simulink model "generic_truck"  (R2025a)
settings: Solver=VariableStepAuto  StartTime=0.0  StopTime=600  FixedStep=0.01  MaxStep=0.001  RelTol=1e-3  EnableMultiTasking=on
libraries: TruckMaker4SL x205, simulink x1
(part 1 of 9)
settings Model: ModifiedByFormat=IPG  SimulationMode=accelerator  NumberOfSteps=10  ExtModeAutoUpdateStatusClock=off  Creator=IPG  LastModifiedBy=IPG
settings SolverCC: AlgebraicLoopSolver=TrustRegion
settings DataIOCC: LimitDataPoints=on  SaveFormat=Array  SignalLoggingSaveFormat=ModelDataLogs  ReturnWorkspaceOutputs=off  SignalLoggingName=sigsOut
settings OptimizationCC: BooleanDataType=off  ReuseModelBlockBuffer=off  ExpressionDepthLimit=2147483647.0  InitFltsAndDblsToZero=on  LifeSpan=inf
settings DebuggingCC: SaveWithParameterizedLinksMsg=none  UnderspecifiedInitializationDetection=Classic  MergeDetectMultiDrivingBlocksExec=none  SignalResolutionControl=TryResolveAllWithWarning  MultiTaskDSMMsg=warning  MultiTaskCondExecSysMsg=none  FcnCallInpInsideContextMsg=warning  UnconnectedInputMsg=warning  UnconnectedOutputMsg=warning  UnconnectedLineMsg=warning  StateNameClashWarn=warning  SFUnexpectedBacktrackingDiag=warning  SFNoUnconditionalDefaultTransitionDiag=warning  ArithmeticOperatorsInVariantConditions=warning
settings HardwareCC: ProdBitPerPointer=32.0  ProdBitPerSizeT=32.0  ProdBitPerPtrDiffT=32.0  ProdLargestAtomicFloat=None  ProdIntDivRoundTo=Undefined  ProdEndianess=Unspecified  ProdWordSize=32.0  ProdHWDeviceType=32-bit Generic  TargetUnknown=on
settings ModelReferenceCC: EnableRefExpFcnMdlSchedulingChecks=on  PropagateSignalLabelsOutOfModel=off
settings SFSimCC: SimUseLocalCustomCode=off  CustomCodeUndefinedFunction=UseInterfaceOnly
settings RTWCC: RTWUseLocalCustomCode=off  GPUComputeCapability=3.5  DLArmComputeVersion=19.05
settings CodeAppCC: MaxIdLength=63.0  StateflowObjectComments=on
settings GRTTargetCC: TargetFcnLib=ansi_tfl_tmw.mat  TargetLangStandard=C89/C90 (ANSI)  CombineOutputUpdateFcns=off  GRTInterface=on
settings ConfigComp: CovMetricSettings=dw  CovSaveCumulativeToWorkspaceVar=on  CovSaveSingleToWorkspaceVar=on  CovExternalEMLEnable=off

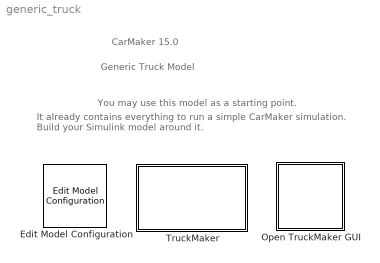
== system generic_truck ==
  note: Generic Truck Model
  note: CarMaker 15.0
  note: You may use this model as a starting point.
  note: It already contains everything to run a simple CarMaker simulation.
      | Build your Simulink model around it.
  Edit Model Configuration : TruckMaker4SL/Edit Model Configuration  SFunctionModules=''
      settings: SourceProductName=TruckMaker4SL
  Open TruckMaker GUI : Subsystem  LoadFcn=if ~length(which('cmself')), cmenv; end
      settings: OpenFcn=cmblockmagic('gui_fix_display'); TM_Simulink
      mask Display: image(imread('TruckMakerGUI.png'));
  TruckMaker : Subsystem  TreatAsAtomicUnit=on
      mask Display: image(imread('TruckMakerSys.png'));

== system generic_truck/Open TruckMaker GUI ==
  S-Function : S-Function  FunctionName=cm_gui  SFunctionDeploymentMode=off  EnableBusSupport=off

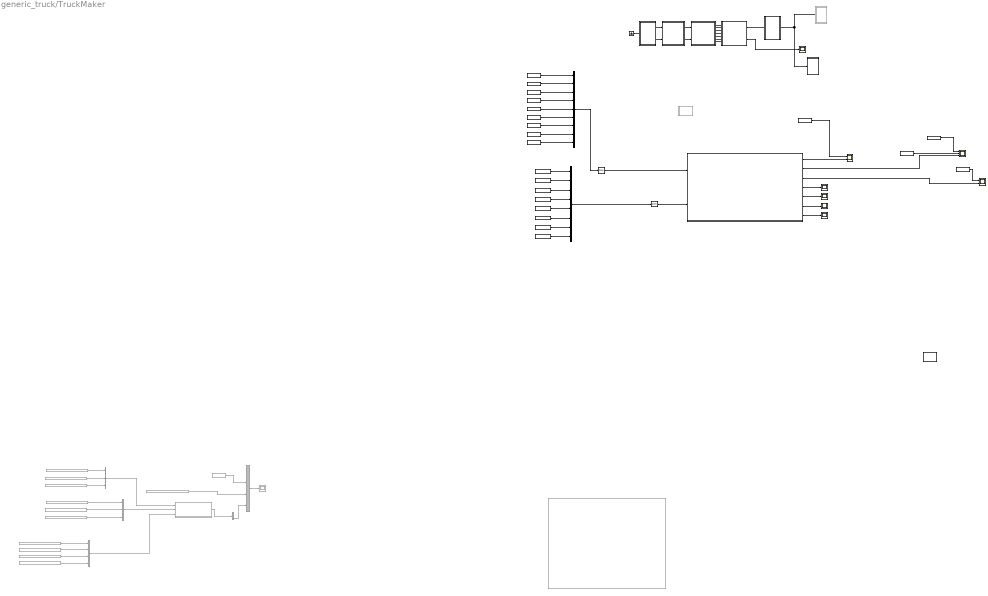
== system generic_truck/TruckMaker ==
  ACC_X : TruckMaker4SL/Read CM Dict  xname=Sensor.Inertial.Vhcl.VchBdy.Acc_B.x  xsync=off  xstime=Continuous
      settings: SourceProductName=TruckMaker4SL
  ACC_Y : TruckMaker4SL/Read CM Dict  xname=Sensor.Inertial.Vhcl.VchBdy.Acc_B.y  xsync=off  xstime=Continuous
      settings: SourceProductName=TruckMaker4SL
  CM_FIRST : Subsystem
  CM_LAST : Subsystem
  "Comparison Block Forces " : Subsystem  Commented=on
  CyFL : Scope
      settings: ActiveDisplayYMinimum=3.9269565785362603  ActiveDisplayYMaximum=4.6568214685506568  DataLoggingVariableName=ScopeData4
  CyFR : Scope
      settings: ActiveDisplayYMinimum=3.9070435148857565  ActiveDisplayYMaximum=4.836023488585889  DataLoggingVariableName=ScopeData9
  CyRL : Scope
      settings: ActiveDisplayYMinimum=3.932725959975766  ActiveDisplayYMaximum=4.6054934360163191  DataLoggingVariableName=ScopeData20
  CyRR : Scope
      settings: ActiveDisplayYMinimum=3.9355217806460492  ActiveDisplayYMaximum=4.5803309951451876  DataLoggingVariableName=ScopeData21
  Demux4 : Demux  Commented=on  Outputs=2
  DrivMan : Subsystem
  Ground : Ground
  IPG Vehicle : Subsystem  TreatAsAtomicUnit=on
  MATLAB Function : MATLAB Function  TreatAsAtomicUnit=on
  MATLAB Function1 : MATLAB Function  Commented=on  TreatAsAtomicUnit=on
  Mux : Mux  Inputs=9
  Mux20 : Mux  Commented=on
  Mux21 : Mux  Commented=on
  Mux22 : Mux  Commented=on  Inputs=3
  Mux24 : Mux  Inputs=8
  Mux5 : Mux  Commented=on  Inputs=3
  OMEGA_Z : TruckMaker4SL/Read CM Dict  xname=Car.YawRate  xsync=off  xstime=Continuous
      settings: SourceProductName=TruckMaker4SL
  OMEGA_Z1 : TruckMaker4SL/Read CM Dict  xname=Vhcl.YawRate  xsync=off  xstime=Continuous
      settings: SourceProductName=TruckMaker4SL
  Read CM Dict : TruckMaker4SL/Read CM Dict  xname=Car.vx  xsync=off  xstime=Continuous
      settings: SourceProductName=TruckMaker4SL
  Read CM Dict1 : TruckMaker4SL/Read CM Dict  xname=Vhcl.RL.Trq_Drive  xsync=off  xstime=Continuous
      settings: SourceProductName=TruckMaker4SL
  Read CM Dict10 : TruckMaker4SL/Read CM Dict  xname=Vhcl.FL.Trq_Drive  xsync=off  xstime=Continuous
      settings: SourceProductName=TruckMaker4SL
  Read CM Dict2 : TruckMaker4SL/Read CM Dict  xname=Vhcl.FR.Trq_Drive  xsync=off  xstime=Continuous
      settings: SourceProductName=TruckMaker4SL
  Read CM Dict3 : TruckMaker4SL/Read CM Dict  xname=Car.SteerAngleRL  xsync=off  xstime=Continuous
      settings: SourceProductName=TruckMaker4SL
  Read CM Dict4 : TruckMaker4SL/Read CM Dict  xname=Car.vy  xsync=off  xstime=Continuous
      settings: SourceProductName=TruckMaker4SL
  Read CM Dict5 : TruckMaker4SL/Read CM Dict  xname=Car.SteerAngleFR  xsync=off  xstime=Continuous
      settings: SourceProductName=TruckMaker4SL
  Read CM Dict7 : TruckMaker4SL/Read CM Dict  xname=Car.SteerAngleRR  xsync=off  xstime=Continuous
      settings: SourceProductName=TruckMaker4SL
  Read CM Dict8 : TruckMaker4SL/Read CM Dict  xname=Vhcl.RR.Trq_Drive  xsync=off  xstime=Continuous
      settings: SourceProductName=TruckMaker4SL
  Read CM Dict9 : TruckMaker4SL/Read CM Dict  xname=Car.SteerAngleFL  xsync=off  xstime=Continuous
      settings: SourceProductName=TruckMaker4SL
  Scope1 : Scope
      settings: ActiveDisplayYMinimum=-1868.760709207141  ActiveDisplayYMaximum=1405.9236144331162
  Scope9 : Scope  Commented=on
      settings: ActiveDisplayYMinimum=-0.65921669576004926  ActiveDisplayYMaximum=0.79450479585309486  DataLoggingVariableName=ScopeData22
  Sensor_Vx : TruckMaker4SL/Read CM Dict  xname=Sensor.Inertial.Vhcl.VchBdy.Vel_B.x  xsync=off  xstime=Continuous
      settings: SourceProductName=TruckMaker4SL
  Sensor_Vy : TruckMaker4SL/Read CM Dict  xname=Sensor.Inertial.Vhcl.VchBdy.Vel_B.y  xsync=off  xstime=Continuous
      settings: SourceProductName=TruckMaker4SL
  Sensor_Vy1 : TruckMaker4SL/Read CM Dict  xname=Sensor.Inertial.Vhcl.VchBdy.Vel_B.y  xsync=off  xstime=Continuous
      settings: SourceProductName=TruckMaker4SL
  Subsystem1 : Subsystem  Commented=on
  "Tractor_Subsystem " : Subsystem
  Two_TRack_Model : Subsystem
  UKF_Articulated_Vehicles : MATLAB Function  Commented=on  TreatAsAtomicUnit=on
  VehicleControl : Subsystem
  Vx : Scope  NumInputPorts=2
      settings: ActiveDisplayYMinimum=-2.172157780455624  ActiveDisplayYMaximum=19.549373141935231  DataLoggingVariableName=ScopeData6
  Vy : Scope  NumInputPorts=3
      settings: ActiveDisplayYMinimum=-0.96685371412713816  ActiveDisplayYMaximum=0.99853922756367719  DataLoggingVariableName=ScopeData3
  Vy_FL_sen3 : TruckMaker4SL/Read CM Dict  Commented=on  xname=Car.vyFL  xsync=off  xstime=Continuous
      settings: SourceProductName=TruckMaker4SL
  Wz : Scope  NumInputPorts=2
      settings: ActiveDisplayYMinimum=-0.034454715390692593  ActiveDisplayYMaximum=0.28039320476498558  DataLoggingVariableName=ScopeData10
  Zero-Order Hold : ZeroOrderHold  SampleTime=0.01
  Zero-Order Hold1 : ZeroOrderHold  SampleTime=0.01
  omegaRL : TruckMaker4SL/Read CM Dict  xname=Vhcl.RL.rotv  xsync=off  xstime=Continuous
      settings: SourceProductName=TruckMaker4SL
  omegaRR : TruckMaker4SL/Read CM Dict  xname=Vhcl.RR.rotv  xsync=off  xstime=Continuous
      settings: SourceProductName=TruckMaker4SL
  omegaTireFL : TruckMaker4SL/Read CM Dict  xname=Vhcl.FL.rotv  xsync=off  xstime=Continuous
      settings: SourceProductName=TruckMaker4SL
  omegaTireFR : TruckMaker4SL/Read CM Dict  xname=Vhcl.FR.rotv  xsync=off  xstime=Continuous
      settings: SourceProductName=TruckMaker4SL
  wx10 : TruckMaker4SL/Read CM Dict  Commented=on  xname=Sensor.Inertial.Vhcl.VchBdy.Omega_B.z  xsync=off  xstime=Continuous
      settings: SourceProductName=TruckMaker4SL
  wx3 : TruckMaker4SL/Read CM Dict  Commented=on  xname=Car.vx  xsync=off  xstime=Continuous
      settings: SourceProductName=TruckMaker4SL
  wx4 : TruckMaker4SL/Read CM Dict  Commented=on  xname=Car.CamberFL  xsync=off  xstime=Continuous
      settings: SourceProductName=TruckMaker4SL
  wx5 : TruckMaker4SL/Read CM Dict  Commented=on  xname=Car.vy  xsync=off  xstime=Continuous
      settings: SourceProductName=TruckMaker4SL
  wx6 : TruckMaker4SL/Read CM Dict  Commented=on  xname=Car.vz  xsync=off  xstime=Continuous
      settings: SourceProductName=TruckMaker4SL
  wx7 : TruckMaker4SL/Read CM Dict  Commented=on  xname=Sensor.Inertial.Vhcl.FL.Vel_B.y  xsync=off  xstime=Continuous
      settings: SourceProductName=TruckMaker4SL
  wx8 : TruckMaker4SL/Read CM Dict  Commented=on  xname=Sensor.Inertial.Vhcl.VchBdy.Omega_B.x  xsync=off  xstime=Continuous
      settings: SourceProductName=TruckMaker4SL
  wx9 : TruckMaker4SL/Read CM Dict  Commented=on  xname=Sensor.Inertial.Vhcl.VchBdy.Omega_B.y  xsync=off  xstime=Continuous
      settings: SourceProductName=TruckMaker4SL
  wy4 : TruckMaker4SL/Read CM Dict  Commented=on  xname=Car.CamberFR  xsync=off  xstime=Continuous
      settings: SourceProductName=TruckMaker4SL
  wz8 : TruckMaker4SL/Read CM Dict  Commented=on  xname=Car.CamberRL  xsync=off  xstime=Continuous
      settings: SourceProductName=TruckMaker4SL
  wz9 : TruckMaker4SL/Read CM Dict  Commented=on  xname=Car.CamberRR  xsync=off  xstime=Continuous
      settings: SourceProductName=TruckMaker4SL
  wires:
  VehicleControl/2(Vhcl.Model.Source) -> IPG Vehicle/2(Vhcl.Model.Source)
  VehicleControl/7(VhclCtrl.PT) -> IPG Vehicle/7(VhclCtrl.PT)
  VehicleControl/6(VhclCtrl.Brake) -> IPG Vehicle/6(VhclCtrl.Brake)
  VehicleControl/5(Vhcl.Misc) -> IPG Vehicle/5(Vhcl.Misc)
  VehicleControl/4(Vhcl.Wheel.In) -> IPG Vehicle/4(Vhcl.Wheel.In)
  VehicleControl/3(VhclCtrl.Steering) -> IPG Vehicle/3(VhclCtrl.Steering)
  VehicleControl/1(Sync_Out) -> IPG Vehicle/1(Sync_In)
  IPG Vehicle/1(Sync_Out) -> CM_LAST/1(Sync_In)
  Ground/1 -> CM_FIRST/1(Sync_In)
  CM_LAST/1(Sync_Out) -> Subsystem1/1(Sync), "Tractor_Subsystem "/1(Sync)
  CM_FIRST/1(Sync_Out) -> DrivMan/1(Sync_In)
  CM_FIRST/2(Env.Misc) -> DrivMan/2(Env.Misc)
  DrivMan/1(Sync_Out) -> VehicleControl/1(Sync_In)
  DrivMan/2(DrivMan.Out) -> VehicleControl/2(DrivMan.In)
  IPG Vehicle/2(WRR_Trq-drive) -> Scope1/1
  ACC_X/1 -> Mux/1
  Two_TRack_Model/2(vy) -> Vy/3  "estimated_vhl_vy"
  Two_TRack_Model/4(CyFL) -> CyFL/1  "CyFL"
  Sensor_Vx/1 -> Mux/3
  Sensor_Vy/1 -> Mux/4
  OMEGA_Z/1 -> Mux/5  "omega_sensor"
  Two_TRack_Model/1(vx) -> Vx/2  "estimated_vhl_vx"
  Two_TRack_Model/3(wz) -> Wz/2  "estimated_vhl_wz"
  ACC_Y/1 -> Mux/2
  wz9/1 -> Mux21/4
  wx4/1 -> Mux21/1
  wy4/1 -> Mux21/2
  wz8/1 -> Mux21/3
  MATLAB Function1/1(V_FL) -> Demux4/1
  Mux20/1 -> Scope9/1
  wx3/1 -> Mux22/1
  wx6/1 -> Mux22/3
  wx5/1 -> Mux22/2
  Mux22/1 -> MATLAB Function1/1(CarVelocity)
  Demux4/2 -> Mux20/4
  Vy_FL_sen3/1 -> Mux20/2  "CAR_VyFL"
  wx7/1 -> Mux20/3  "sensor_wheelCenter"
  wx8/1 -> Mux5/1
  Read CM Dict7/1 -> Mux24/4
  Read CM Dict3/1 -> Mux24/3
  Read CM Dict5/1 -> Mux24/2
  Read CM Dict9/1 -> Mux24/1
  Mux24/1 -> Zero-Order Hold1/1
  Mux/1 -> Zero-Order Hold/1
  wx9/1 -> Mux5/2
  wx10/1 -> Mux5/3
  Mux5/1 -> MATLAB Function1/2(CarOmega)
  Mux21/1 -> MATLAB Function1/3(WheelCamberAngle)
  omegaTireFL/1 -> Mux/6  "omegaTireFL"
  omegaTireFR/1 -> Mux/7  "omegaTireFR"
  omegaRL/1 -> Mux/8  "omegaTireRL"
  omegaRR/1 -> Mux/9  "omegaTireRR"
  Read CM Dict10/1 -> Mux24/5
  Read CM Dict2/1 -> Mux24/6
  Read CM Dict1/1 -> Mux24/7
  Read CM Dict8/1 -> Mux24/8
  Read CM Dict/1 -> Vx/1
  Read CM Dict4/1 -> Vy/1
  Sensor_Vy1/1 -> Vy/2
  OMEGA_Z1/1 -> Wz/1  "omega_sensor"
  Two_TRack_Model/7(CyFR) -> CyRR/1  "CyRR"
  Two_TRack_Model/6(CyRR) -> CyRL/1  "CyRL"
  Two_TRack_Model/5(CyRL) -> CyFR/1  "CyFR"
  Zero-Order Hold/1 -> Two_TRack_Model/1(Mesurement)
  Zero-Order Hold1/1 -> Two_TRack_Model/2(Inputs)

== system generic_truck/TruckMaker/CM_FIRST ==
  Sync_In : Inport
  BusCreator1 : BusCreator  Inputs=8
  BusCreator2 : BusCreator  Inputs=6
  Demux1 : Demux  Outputs=14
      settings: DisplayOption=none
  Environment : S-Function  FunctionName=TM_Sfun  Parameters='Environment'  SFunctionDeploymentMode=off  EnableBusSupport=off
  IoIn : S-Function  FunctionName=TM_Sfun  Parameters='IoIn'  SFunctionDeploymentMode=off  EnableBusSupport=off
  Terminator : Terminator
  Sync_Out : Outport  VectorParamsAs1DForOutWhenUnconnected=off
  Env.Misc : Outport  Port=2  VectorParamsAs1DForOutWhenUnconnected=off
  wires:
  BusCreator2/1 -> Terminator/1  "IF Environment (in)"
  BusCreator1/1 -> Env.Misc/1
  Demux1/14 -> BusCreator2/6  "Env sRoad"
  Demux1/13 -> BusCreator2/5  "Env PoI_GCS Elev"
  Demux1/12 -> BusCreator2/4  "Env PoI_GCS Lat"
  Demux1/11 -> BusCreator2/3  "Env PoI_GCS Long"
  Demux1/10 -> BusCreator2/2  "Env Time"
  Demux1/9 -> BusCreator2/1  "Env yDay"
  Demux1/8 -> BusCreator1/8  "Env WindVel_tot z"
  Demux1/7 -> BusCreator1/7  "Env WindVel_tot y"
  Demux1/6 -> BusCreator1/6  "Env WindVel_tot x"
  Demux1/5 -> BusCreator1/5  "Env SolarRadiation"
  Demux1/4 -> BusCreator1/4  "Env AirHumidity"
  Demux1/3 -> BusCreator1/3  "Env AirPressure"
  Demux1/2 -> BusCreator1/2  "Env AirDensity"
  Demux1/1 -> BusCreator1/1  "Env Temperature"
  Environment/2 -> Demux1/1
  Environment/1 -> Sync_Out/1
  IoIn/1 -> Environment/1
  Sync_In/1 -> IoIn/1

== system generic_truck/TruckMaker/CM_LAST ==
  Sync_In : Inport
  CM_User : S-Function  FunctionName=TM_Sfun  Parameters='CM_User'  SFunctionDeploymentMode=off  EnableBusSupport=off
  IoOut : S-Function  FunctionName=TM_Sfun  Parameters='IoOut'  SFunctionDeploymentMode=off  EnableBusSupport=off
  Sync_Out : Outport  VectorParamsAs1DForOutWhenUnconnected=off
  wires:
  IoOut/1 -> Sync_Out/1
  CM_User/1 -> IoOut/1
  Sync_In/1 -> CM_User/1

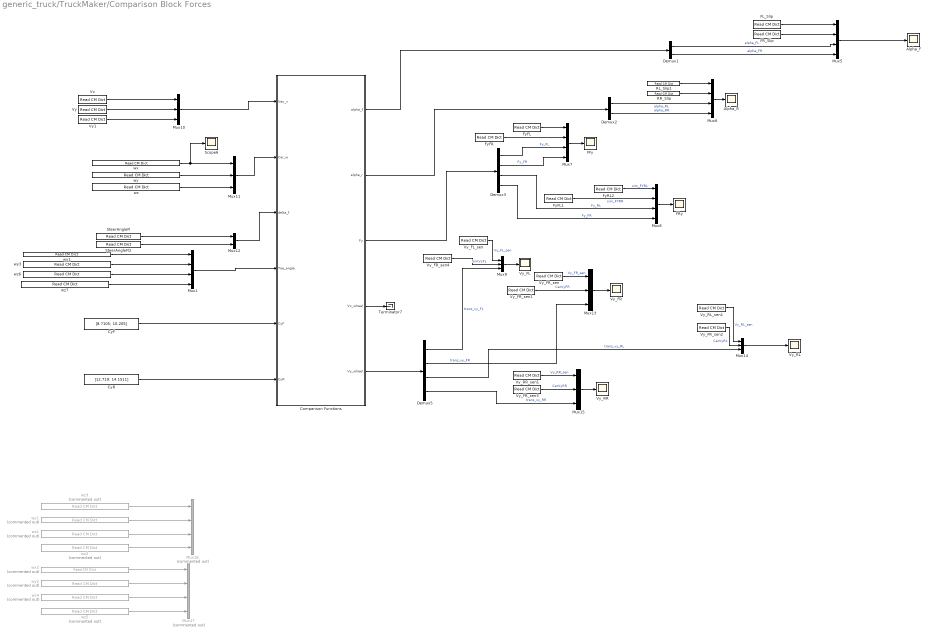
== system generic_truck/TruckMaker/Comparison Block Forces  ==
  Alpha_F : Scope
      settings: ActiveDisplayYMinimum=-0.021004916867085378  ActiveDisplayYMaximum=0.0090064384954623433  DataLoggingVariableName=ScopeData11
  Alpha_R : Scope
      settings: ActiveDisplayYMinimum=-0.023492270502238927  ActiveDisplayYMaximum=-0.021229702307656122  DataLoggingVariableName=ScopeData12
  "Comparison Functions " : MATLAB Function  TreatAsAtomicUnit=on
  CyF : Constant  Value=[8.7105; 10.205]
  CyR : Constant  Value=[12.719; 14.1511]
  Demux1 : Demux  Outputs=2
  Demux2 : Demux  Outputs=2
  Demux3 : Demux
  Demux5 : Demux
  FFy : Scope
      settings: ActiveDisplayYMinimum=-11443.527316616819  ActiveDisplayYMaximum=22637.438313337225  DataLoggingVariableName=ScopeData13
  FL_Slip : TruckMaker4SL/Read CM Dict  xname=Vhcl.FL.SideSlip  xsync=off  xstime=Continuous
      settings: SourceProductName=TruckMaker4SL
  FR_Slip : TruckMaker4SL/Read CM Dict  xname=Vhcl.FR.SideSlip  xsync=off  xstime=Continuous
      settings: SourceProductName=TruckMaker4SL
  FRy : Scope
      settings: ActiveDisplayYMinimum=-853.982895939768  ActiveDisplayYMaximum=3729.98380628211  DataLoggingVariableName=ScopeData14
  FyFL : TruckMaker4SL/Read CM Dict  xname=Car.FyFL  xsync=off  xstime=Continuous
      settings: SourceProductName=TruckMaker4SL
  FyFL1 : TruckMaker4SL/Read CM Dict  xname=Vhcl.RR.Fy  xsync=off  xstime=Continuous
      settings: SourceProductName=TruckMaker4SL
  FyFR : TruckMaker4SL/Read CM Dict  xname=Car.FyFR  xsync=off  xstime=Continuous
      settings: SourceProductName=TruckMaker4SL
  FyRL2 : TruckMaker4SL/Read CM Dict  xname=Vhcl.RL.Fy  xsync=off  xstime=Continuous
      settings: SourceProductName=TruckMaker4SL
  Mux{1,5..8} (5 alike) : Mux
  Mux{9..11,13..15} (6 alike) : Mux  Inputs=3
  Mux12 : Mux  Inputs=2
  Mux16 : Mux  Commented=on
  Mux17 : Mux  Commented=on
  RL_Slip1 : TruckMaker4SL/Read CM Dict  xname=Vhcl.RL.SideSlip  xsync=off  xstime=Continuous
      settings: SourceProductName=TruckMaker4SL
  RR_Slip : TruckMaker4SL/Read CM Dict  xname=Vhcl.RR.SideSlip  xsync=off  xstime=Continuous
      settings: SourceProductName=TruckMaker4SL
  Scope6 : Scope
      settings: ActiveDisplayYMinimum=-0.0026761211979278751  ActiveDisplayYMaximum=0.00092040105898752271  DataLoggingVariableName=ScopeData19
  SteerAngleFl : TruckMaker4SL/Read CM Dict  xname=Car.SteerAngleFL  xsync=off  xstime=Continuous
      settings: SourceProductName=TruckMaker4SL
  SteerAngleFl2 : TruckMaker4SL/Read CM Dict  xname=Car.SteerAngleFR  xsync=off  xstime=Continuous
      settings: SourceProductName=TruckMaker4SL
  Terminator7 : Terminator
  Vx : TruckMaker4SL/Read CM Dict  xname=Car.vx  xsync=off  xstime=Continuous
      settings: SourceProductName=TruckMaker4SL
  Vy : TruckMaker4SL/Read CM Dict  xname=Car.vy  xsync=off  xstime=Continuous
      settings: SourceProductName=TruckMaker4SL
  Vy1 : TruckMaker4SL/Read CM Dict  xname=Car.vz  xsync=off  xstime=Continuous
      settings: SourceProductName=TruckMaker4SL
  Vy_FL : Scope
      settings: ActiveDisplayYMinimum=-0.57174357690667166  ActiveDisplayYMaximum=-0.56027134618639107  DataLoggingVariableName=ScopeData15
  Vy_FL_sen : TruckMaker4SL/Read CM Dict  xname=Sensor.Inertial.Vhcl.FL.Vel_B.y  xsync=off  xstime=Continuous
      settings: SourceProductName=TruckMaker4SL
  Vy_FR : Scope
      settings: ActiveDisplayYMinimum=-0.69251799128236324  ActiveDisplayYMaximum=0.38771666797496468  DataLoggingVariableName=ScopeData16
  Vy_FR_sen : TruckMaker4SL/Read CM Dict  xname=Sensor.Inertial.Vhcl.FR.Vel_B.y  xsync=off  xstime=Continuous
      settings: SourceProductName=TruckMaker4SL
  Vy_FR_sen1 : TruckMaker4SL/Read CM Dict  xname=Car.vyFR  xsync=off  xstime=Continuous
      settings: SourceProductName=TruckMaker4SL
  Vy_FR_sen2 : TruckMaker4SL/Read CM Dict  xname=Car.vyRL  xsync=off  xstime=Continuous
      settings: SourceProductName=TruckMaker4SL
  Vy_FR_sen3 : TruckMaker4SL/Read CM Dict  xname=Car.vyRR  xsync=off  xstime=Continuous
      settings: SourceProductName=TruckMaker4SL
  Vy_FR_sen4 : TruckMaker4SL/Read CM Dict  xname=Car.vyFL  xsync=off  xstime=Continuous
      settings: SourceProductName=TruckMaker4SL
  Vy_RL : Scope
      settings: ActiveDisplayYMinimum=-0.44354593338472575  ActiveDisplayYMaximum=-0.3528419695854797  DataLoggingVariableName=ScopeData17
  Vy_RL_sen1 : TruckMaker4SL/Read CM Dict  xname=Sensor.Inertial.Vhcl.RL.Vel_B.y  xsync=off  xstime=Continuous
      settings: SourceProductName=TruckMaker4SL
  Vy_RR : Scope
      settings: ActiveDisplayYMinimum=-0.39718843046100355  ActiveDisplayYMaximum=-0.37307460740982057  DataLoggingVariableName=ScopeData18
  Vy_RR_sen1 : TruckMaker4SL/Read CM Dict  xname=Sensor.Inertial.Vhcl.RR.Vel_B.y  xsync=off  xstime=Continuous
      settings: SourceProductName=TruckMaker4SL
  wx : TruckMaker4SL/Read CM Dict  xname=Sensor.Inertial.Vhcl.VchBdy.Omega_B.x  xsync=off  xstime=Continuous
      settings: SourceProductName=TruckMaker4SL
  wx1 : TruckMaker4SL/Read CM Dict  xname=Car.ToeFL  xsync=off  xstime=Continuous
      settings: SourceProductName=TruckMaker4SL
  wx2 : TruckMaker4SL/Read CM Dict  Commented=on  xname=Car.CamberFL  xsync=off  xstime=Continuous
      settings: SourceProductName=TruckMaker4SL
  wy : TruckMaker4SL/Read CM Dict  xname=Sensor.Inertial.Vhcl.VchBdy.Omega_B.y  xsync=off  xstime=Continuous
      settings: SourceProductName=TruckMaker4SL
  wy1 : TruckMaker4SL/Read CM Dict  Commented=on  xname=Car.InclinAngleFR  xsync=off  xstime=Continuous
      settings: SourceProductName=TruckMaker4SL
  wy2 : TruckMaker4SL/Read CM Dict  Commented=on  xname=Car.CamberFR  xsync=off  xstime=Continuous
      settings: SourceProductName=TruckMaker4SL
  wy3 : TruckMaker4SL/Read CM Dict  xname=Car.ToeFR  xsync=off  xstime=Continuous
      settings: SourceProductName=TruckMaker4SL
  wz : TruckMaker4SL/Read CM Dict  xname=Sensor.Inertial.Vhcl.VchBdy.Omega_B.z  xsync=off  xstime=Continuous
      settings: SourceProductName=TruckMaker4SL
  wz1 : TruckMaker4SL/Read CM Dict  Commented=on  xname=Car.InclinAngleRL  xsync=off  xstime=Continuous
      settings: SourceProductName=TruckMaker4SL
  wz2 : TruckMaker4SL/Read CM Dict  Commented=on  xname=Car.InclinAngleRR  xsync=off  xstime=Continuous
      settings: SourceProductName=TruckMaker4SL
  wz3 : TruckMaker4SL/Read CM Dict  Commented=on  xname=Car.InclinAngleFL  xsync=off  xstime=Continuous
      settings: SourceProductName=TruckMaker4SL
  wz4 : TruckMaker4SL/Read CM Dict  Commented=on  xname=Car.CamberRL  xsync=off  xstime=Continuous
      settings: SourceProductName=TruckMaker4SL
  wz5 : TruckMaker4SL/Read CM Dict  Commented=on  xname=Car.CamberRR  xsync=off  xstime=Continuous
      settings: SourceProductName=TruckMaker4SL
  wz6 : TruckMaker4SL/Read CM Dict  xname=Car.ToeRL  xsync=off  xstime=Continuous
      settings: SourceProductName=TruckMaker4SL
  wz7 : TruckMaker4SL/Read CM Dict  xname=Car.ToeRR  xsync=off  xstime=Continuous
      settings: SourceProductName=TruckMaker4SL
  wires:
  Vy/1 -> Mux10/2
  Mux14/1 -> Vy_RL/1
  Vx/1 -> Mux10/1
  Demux5/4 -> Mux15/3  "trans_vy_RR"
  Mux8/1 -> FRy/1
  FyFL1/1 -> Mux8/2  "sim_FYRR"
  Demux3/4 -> Mux8/4  "Fy_FR"
  Mux11/1 -> "Comparison Functions "/2(Car_w)
  RL_Slip1/1 -> Mux6/1
  Mux6/1 -> Alpha_R/1
  RR_Slip/1 -> Mux6/2
  Mux9/1 -> Vy_FL/1
  Mux13/1 -> Vy_FR/1
  wz2/1 -> Mux16/4
  wx/1 -> Scope6/1, Mux11/1
  Mux15/1 -> Vy_RR/1
  Vy_RL_sen1/1 -> Mux14/1  "Vy_RL_sen"
  FyFR/1 -> Mux7/2
  FyRL2/1 -> Mux8/1  "sim_FYRL"
  CyF/1 -> "Comparison Functions "/5(CyF)
  Mux7/1 -> FFy/1
  Mux5/1 -> Alpha_F/1
  FyFL/1 -> Mux7/1
  FR_Slip/1 -> Mux5/2
  "Comparison Functions "/2(alpha_r) -> Demux2/1
  wx2/1 -> Mux17/1
  Demux5/2 -> Mux13/3  "trans_vy_FR"
  Vy_FR_sen/1 -> Mux13/1  "Vy_FR_sen"
  FL_Slip/1 -> Mux5/1
  Mux12/1 -> "Comparison Functions "/3(delta_f)
  "Comparison Functions "/3(Fy) -> Demux3/1
  wz3/1 -> Mux16/1
  SteerAngleFl/1 -> Mux12/1
  Vy1/1 -> Mux10/3
  Demux3/1 -> Mux7/3  "Fy_FL"
  wy1/1 -> Mux16/2
  "Comparison Functions "/4(Vx_wheel) -> Terminator7/1
  "Comparison Functions "/5(Vy_wheel) -> Demux5/1
  Vy_RR_sen1/1 -> Mux15/1  "Vy_RR_sen"
  Demux5/1 -> Mux9/3  "trans_vy_FL"
  SteerAngleFl2/1 -> Mux12/2
  Demux3/2 -> Mux7/4  "Fy_FR"
  CyR/1 -> "Comparison Functions "/6(CyR)
  "Comparison Functions "/1(alpha_f) -> Demux1/1
  wz4/1 -> Mux17/3
  Mux10/1 -> "Comparison Functions "/1(Vec_v)
  Demux2/2 -> Mux6/4  "alpha_RR"
  Demux2/1 -> Mux6/3  "alpha_RL"
  Vy_FL_sen/1 -> Mux9/1  "Vy_FL_sen"
  Demux3/3 -> Mux8/3  "Fy_RL"
  wy2/1 -> Mux17/2
  wz5/1 -> Mux17/4
  wz1/1 -> Mux16/3
  wy/1 -> Mux11/2
  wz/1 -> Mux11/3
  Demux5/3 -> Mux14/3  "trans_vy_RL"
  Demux1/2 -> Mux5/4  "alpha_FR"
  Demux1/1 -> Mux5/3  "alpha_FL"
  Vy_FR_sen1/1 -> Mux13/2  "CarVyFR"
  Vy_FR_sen2/1 -> Mux14/2  "CarVyRL"
  Vy_FR_sen3/1 -> Mux15/2  "CarVyRR"
  Vy_FR_sen4/1 -> Mux9/2  "SimVyFL"
  wz6/1 -> Mux1/3
  wy3/1 -> Mux1/2
  wx1/1 -> Mux1/1
  Mux1/1 -> "Comparison Functions "/4(Toe_angle)
  wz7/1 -> Mux1/4

== system generic_truck/TruckMaker/DrivMan ==
  note: There's rarely a reason to override DrivMan signals.
      | Use the VehicleControl interface for this purpose.
  Sync_In : Inport
  Env.Misc : Inport  Port=2
  BusCreator : BusCreator  Inputs=20
  Demux : Demux  Outputs=20
      settings: DisplayOption=none
  DrivMan : S-Function  FunctionName=TM_Sfun  Parameters='DrivMan'  SFunctionDeploymentMode=off  EnableBusSupport=off
  Sync_Out : Outport  VectorParamsAs1DForOutWhenUnconnected=off
  DrivMan.Out : Outport  Port=2  VectorParamsAs1DForOutWhenUnconnected=off
  wires:
  Demux/8 -> BusCreator/8  "DrivMan SelectorCtrl"
  Demux/7 -> BusCreator/7  "DrivMan UserSignal4"
  Demux/6 -> BusCreator/6  "DrivMan UserSignal3"
  Demux/5 -> BusCreator/5  "DrivMan UserSignal2"
  Demux/4 -> BusCreator/4  "DrivMan UserSignal1"
  Demux/3 -> BusCreator/3  "DrivMan UserSignal0"
  Demux/2 -> BusCreator/2  "DrivMan Key"
  Demux/1 -> BusCreator/1  "DrivMan SST"
  Env.Misc/1 -> DrivMan/2
  Sync_In/1 -> DrivMan/1
  DrivMan/1 -> Sync_Out/1
  BusCreator/1 -> DrivMan.Out/1
  DrivMan/2 -> Demux/1
  Demux/9 -> BusCreator/9  "DrivMan DigitalSelectorCtrl0"
  Demux/10 -> BusCreator/10  "DrivMan DigitalSelectorCtrl1"
  Demux/11 -> BusCreator/11  "DrivMan DigitalSelectorCtrl2"
  Demux/20 -> BusCreator/20  "DrivMan Steering Trq"
  Demux/19 -> BusCreator/19  "DrivMan Steering AngAcc"
  Demux/18 -> BusCreator/18  "DrivMan Steering AngVel"
  Demux/17 -> BusCreator/17  "DrivMan Steering Ang"
  Demux/16 -> BusCreator/16  "DrivMan Gas"
  Demux/15 -> BusCreator/15  "DrivMan Clutch"
  Demux/14 -> BusCreator/14  "DrivMan BrakePark"
  Demux/13 -> BusCreator/13  "DrivMan Brake"
  Demux/12 -> BusCreator/12  "DrivMan GearNo"

== system generic_truck/TruckMaker/IPG Vehicle ==
  Sync_In : Inport
  Vhcl.Model.Source : Inport  Port=2
  VhclCtrl.Steering : Inport  Port=3
  Vhcl.Wheel.In : Inport  Port=4
  Vhcl.Misc : Inport  Port=5
  VhclCtrl.Brake : Inport  Port=6
  VhclCtrl.PT : Inport  Port=7
  Brake : Subsystem
  CarAndTrailer : Subsystem
  PowerTrain : Subsystem
  Stop Simulation : Stop
  VehicleSource_BuiltIn : simulink/Logic and Bit Operations/Compare To Constant  relop=~=  const=1  OutDataTypeStr=boolean  ZeroCross=off
  Sync_Out : Outport  VectorParamsAs1DForOutWhenUnconnected=off
  WRR_Trq-drive : Outport  Port=2
  wires:
  VhclCtrl.PT/1 -> PowerTrain/3(VhclCtrl.PT)
  Brake/1(Sync_Out) -> PowerTrain/1(Sync_In)
  CarAndTrailer/1(Sync_Out) -> Brake/1(Sync_In)
  CarAndTrailer/2(Brake.IF.In) -> Brake/2(Brake.IF.In)
  VhclCtrl.Brake/1 -> Brake/3(VhclCtrl.Brake)
  PowerTrain/1(Sync_Out) -> Sync_Out/1
  Vhcl.Misc/1 -> CarAndTrailer/4(Vhcl.Misc)
  Vhcl.Wheel.In/1 -> CarAndTrailer/3(Vhcl.Wheel.In)
  VhclCtrl.Steering/1 -> CarAndTrailer/2(VhclCtrl.Steering)
  Sync_In/1 -> CarAndTrailer/1(Sync_In)
  Vhcl.Model.Source/1 -> VehicleSource_BuiltIn/1
  VehicleSource_BuiltIn/1 -> Stop Simulation/1
  Brake/2(Vhcl.Wheel.PT) -> PowerTrain/2(Vhcl.Wheel.PT)
  PowerTrain/2(WRR_Trq-drive) -> WRR_Trq-drive/1

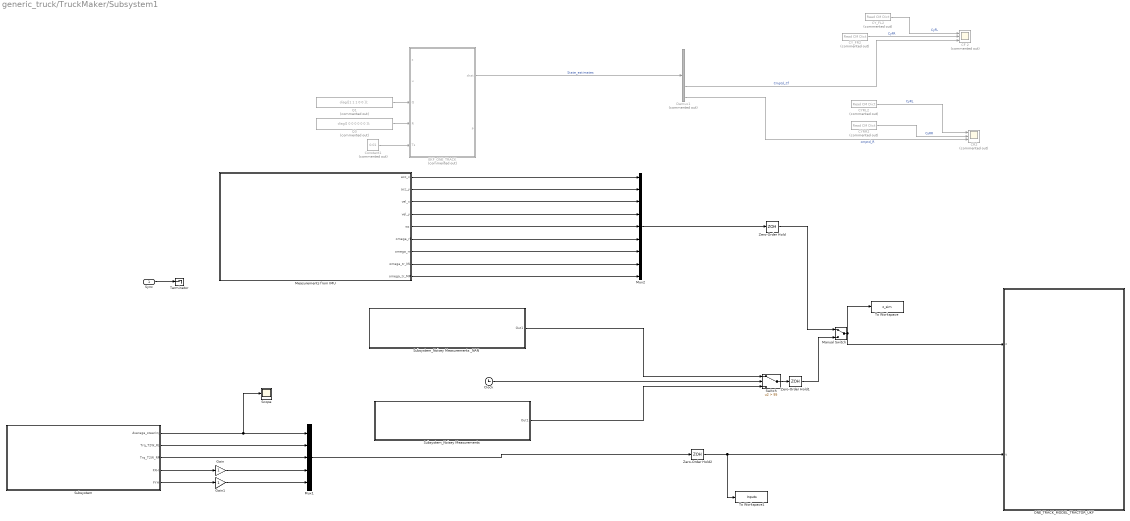
== system generic_truck/TruckMaker/Subsystem1 ==
  Sync : Inport
  CF 2 : Scope  Commented=on  NumInputPorts=3
      settings: ActiveDisplayYMinimum=-74221.220841942573  ActiveDisplayYMaximum=29210.234204256169  DataLoggingVariableName=ScopeData32
  CR2 : Scope  Commented=on  NumInputPorts=3
      settings: ActiveDisplayYMinimum=-5.3363402575311692E+39  ActiveDisplayYMaximum=7.0992603120408667E+38  DataLoggingVariableName=ScopeData33
  CYRL2 : TruckMaker4SL/Read CM Dict  Commented=on  xname=CyRL  xsync=off  xstime=Continuous
      settings: SourceProductName=TruckMaker4SL
  CYRR2 : TruckMaker4SL/Read CM Dict  Commented=on  xname=CyRR  xsync=off  xstime=Continuous
      settings: SourceProductName=TruckMaker4SL
  CY_FL2 : TruckMaker4SL/Read CM Dict  Commented=on  xname=CyFL  xsync=off  xstime=Continuous
      settings: SourceProductName=TruckMaker4SL
  CY_FR2 : TruckMaker4SL/Read CM Dict  Commented=on  xname=CyFR  xsync=off  xstime=Continuous
      settings: SourceProductName=TruckMaker4SL
  Clock : Clock
  Constant1 : Constant  Commented=on  Value=0.01
  Demux1 : Demux  Commented=on  Outputs=5
  EKF_ONE_TRACK : MATLAB Function  Commented=on  TreatAsAtomicUnit=on
  Gain : Gain
  Gain1 : Gain
  Manual Switch : ManualSwitch
  Measurements from IMU : Subsystem  Description=Measurements from IMU Mounted in Vhcl position (3.6; 0.0;1.0)
  Mux1 : Mux  Inputs=5
  Mux2 : Mux  Inputs=9
  ONE_TRACK_MODEL_TRACTOR_UKF : Subsystem
  Q1 : Constant  Commented=on  Value=diag([1 1 1 0 0 ]);
  Q3 : Constant  Commented=on  Value=diag([ 0 0 0 0 0 0 ]);
  Scope : Scope
      settings: ActiveDisplayYMinimum=-0.0066976312723496679  ActiveDisplayYMaximum=0.050256988407650964  DataLoggingVariableName=ScopeData27
  Subsystem : Subsystem
  Subsystem_Noisey Measurements : Subsystem
  Subsystem_Noisey Measurements _NAN : Subsystem
  Switch : Switch  Criteria=u2 > Threshold  Threshold=95  SaturateOnIntegerOverflow=off  InputSameDT=off
  Terminator : Terminator
  To Workspace : ToWorkspace  VariableName=z_sim  SaveFormat=Timeseries  SampleTime=-1
  To Workspace1 : ToWorkspace  VariableName=Inputs  SaveFormat=Timeseries  SampleTime=-1
  Zero-Order Hold : ZeroOrderHold  SampleTime=0.01
  Zero-Order Hold1 : ZeroOrderHold  SampleTime=0.01
  Zero-Order Hold2 : ZeroOrderHold  SampleTime=0.01
  wires:
  Measurements from IMU/3(vel_x) -> Mux2/3
  Mux1/1 -> Zero-Order Hold2/1
  Subsystem/1("Average_steering ") -> Scope/1, Mux1/1
  Subsystem_Noisey Measurements/1(Out1) -> Switch/3
  Q3/1 -> EKF_ONE_TRACK/4(R)
  Q1/1 -> EKF_ONE_TRACK/3(Q)
  Subsystem_Noisey Measurements _NAN/1(Out1) -> Switch/1
  Clock/1 -> Switch/2
  EKF_ONE_TRACK/1(xhat) -> Demux1/1  "State_estimates"
  Subsystem/3(Trq_T2W_RR) -> Mux1/3
  Measurements from IMU/5(wz) -> Mux2/5
  CY_FL2/1 -> CF 2/1  "CyFL"
  CYRR2/1 -> CR2/2  "CyRR"
  Constant1/1 -> EKF_ONE_TRACK/5(Ts)
  Subsystem/2(Trq_T2W_RL) -> Mux1/2
  Measurements from IMU/1(acc_x) -> Mux2/1
  Demux1/4 -> CF 2/3  "Cmptd_Cf"
  CY_FR2/1 -> CF 2/2  "CyFR"
  Measurements from IMU/4(vel_y) -> Mux2/4
  Mux2/1 -> Zero-Order Hold/1
  CYRL2/1 -> CR2/1  "CyRL"
  Measurements from IMU/2(acc_y) -> Mux2/2
  Demux1/5 -> CR2/3  "cmptd_R"
  Manual Switch/1 -> To Workspace/1, ONE_TRACK_MODEL_TRACTOR_UKF/1(z)
  Switch/1 -> Zero-Order Hold1/1
  Sync/1 -> Terminator/1
  Zero-Order Hold/1 -> Manual Switch/1
  Zero-Order Hold1/1 -> Manual Switch/2
  Zero-Order Hold2/1 -> ONE_TRACK_MODEL_TRACTOR_UKF/2(u), To Workspace1/1
  Measurements from IMU/6(omega_rl) -> Mux2/6
  Measurements from IMU/7(omega_rr) -> Mux2/7
  Subsystem/4(FXH) -> Gain/1
  Subsystem/5(FYH) -> Gain1/1
  Measurements from IMU/8(omega_tr_ML) -> Mux2/8
  Measurements from IMU/9(omega_tr_MR) -> Mux2/9
  Gain/1 -> Mux1/4
  Gain1/1 -> Mux1/5

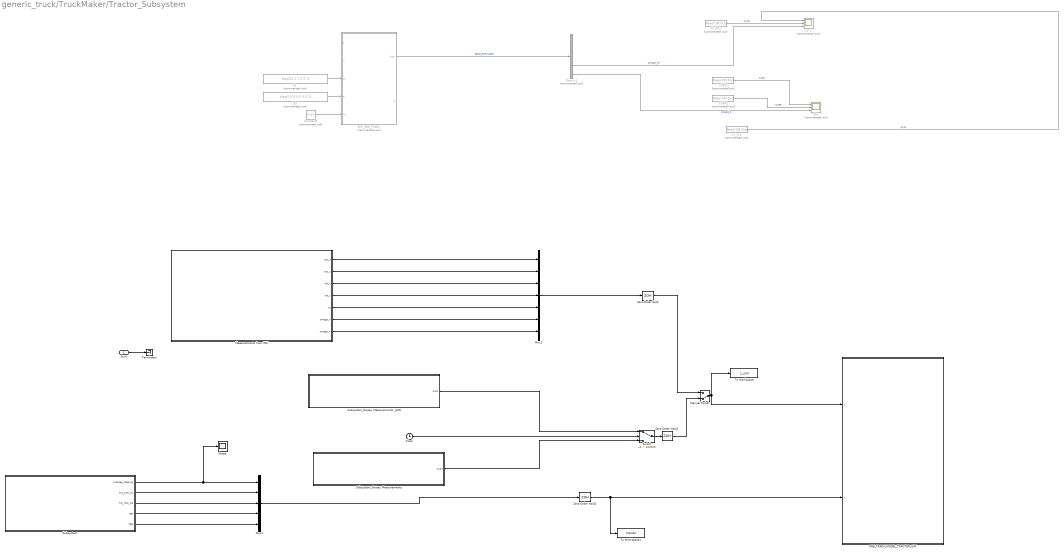
== system generic_truck/TruckMaker/Tractor_Subsystem  ==
  Sync : Inport
  CF 2 : Scope  Commented=on  NumInputPorts=3
      settings: ActiveDisplayYMinimum=-74221.220841942573  ActiveDisplayYMaximum=29210.234204256169  DataLoggingVariableName=ScopeData32
  CR2 : Scope  Commented=on  NumInputPorts=3
      settings: ActiveDisplayYMinimum=-5.3363402575311692E+39  ActiveDisplayYMaximum=7.0992603120408667E+38  DataLoggingVariableName=ScopeData33
  CYRL2 : TruckMaker4SL/Read CM Dict  Commented=on  xname=CyRL  xsync=off  xstime=Continuous
      settings: SourceProductName=TruckMaker4SL
  CYRR2 : TruckMaker4SL/Read CM Dict  Commented=on  xname=CyRR  xsync=off  xstime=Continuous
      settings: SourceProductName=TruckMaker4SL
  CY_FL2 : TruckMaker4SL/Read CM Dict  Commented=on  xname=CyFL  xsync=off  xstime=Continuous
      settings: SourceProductName=TruckMaker4SL
  CY_FR2 : TruckMaker4SL/Read CM Dict  Commented=on  xname=CyFR  xsync=off  xstime=Continuous
      settings: SourceProductName=TruckMaker4SL
  Clock : Clock
  Constant1 : Constant  Commented=on  Value=0.01
  Demux1 : Demux  Commented=on  Outputs=5
  EKF_ONE_TRACK : MATLAB Function  Commented=on  TreatAsAtomicUnit=on
  Manual Switch : ManualSwitch  CurrentSetting=0
  Measurements from IMU : Subsystem  Description=Measurements from IMU Mounted in Vhcl position (3.6; 0.0;1.0)
  Mux1 : Mux  Inputs=5
  Mux2 : Mux  Inputs=7
  ONE_TRACK_MODEL_TRACTOR_UKF : Subsystem
  Q1 : Constant  Commented=on  Value=diag([1 1 1 0 0 ]);
  Q3 : Constant  Commented=on  Value=diag([ 0 0 0 0 0 0 ]);
  Scope : Scope
      settings: ActiveDisplayYMinimum=-0.0066976312723496679  ActiveDisplayYMaximum=0.050256988407650964  DataLoggingVariableName=ScopeData27
  Subsystem : Subsystem
  Subsystem_Noisey Measurements : Subsystem
  Subsystem_Noisey Measurements _NAN : Subsystem
  Switch : Switch  Criteria=u2 > Threshold  Threshold=100000  SaturateOnIntegerOverflow=off  InputSameDT=off
  Terminator : Terminator
  To Workspace : ToWorkspace  VariableName=z_sim  SaveFormat=Timeseries  SampleTime=-1
  To Workspace1 : ToWorkspace  VariableName=Inputs  SaveFormat=Timeseries  SampleTime=-1
  Zero-Order Hold : ZeroOrderHold  SampleTime=0.01
  Zero-Order Hold1 : ZeroOrderHold  SampleTime=0.01
  Zero-Order Hold2 : ZeroOrderHold  SampleTime=0.01
  wires:
  Zero-Order Hold2/1 -> To Workspace1/1, ONE_TRACK_MODEL_TRACTOR_UKF/2(u)
  Zero-Order Hold1/1 -> Manual Switch/2
  Zero-Order Hold/1 -> Manual Switch/1
  Sync/1 -> Terminator/1
  Switch/1 -> Zero-Order Hold1/1
  Manual Switch/1 -> ONE_TRACK_MODEL_TRACTOR_UKF/1(z), To Workspace/1
  Demux1/5 -> CR2/3  "cmptd_R"
  Measurements from IMU/2(acc_y) -> Mux2/2
  CYRL2/1 -> CR2/1  "CyRL"
  Mux2/1 -> Zero-Order Hold/1
  Measurements from IMU/4(vel_y) -> Mux2/4
  CY_FR2/1 -> CF 2/2  "CyFR"
  Demux1/4 -> CF 2/3  "Cmptd_Cf"
  Measurements from IMU/1(acc_x) -> Mux2/1
  Subsystem/2(Trq_T2W_RL) -> Mux1/2
  Constant1/1 -> EKF_ONE_TRACK/5(Ts)
  CYRR2/1 -> CR2/2  "CyRR"
  CY_FL2/1 -> CF 2/1  "CyFL"
  Measurements from IMU/5(wz) -> Mux2/5
  Subsystem/3(Trq_T2W_RR) -> Mux1/3
  EKF_ONE_TRACK/1(xhat) -> Demux1/1  "State_estimates"
  Clock/1 -> Switch/2
  Subsystem_Noisey Measurements _NAN/1(Out1) -> Switch/1
  Q1/1 -> EKF_ONE_TRACK/3(Q)
  Q3/1 -> EKF_ONE_TRACK/4(R)
  Subsystem_Noisey Measurements/1(Out1) -> Switch/3
  Subsystem/1("Average_steering ") -> Scope/1, Mux1/1
  Mux1/1 -> Zero-Order Hold2/1
  Measurements from IMU/3(vel_x) -> Mux2/3
  Measurements from IMU/6(omega_rl) -> Mux2/6
  Measurements from IMU/7(omega_rr) -> Mux2/7
  Subsystem/4(TBF) -> Mux1/4
  Subsystem/5(TBR) -> Mux1/5

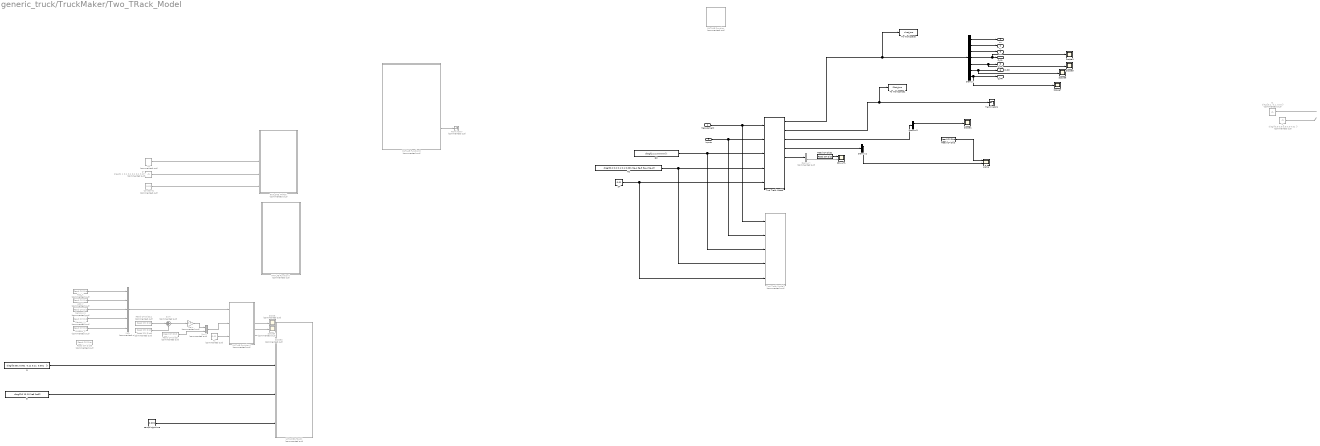
== system generic_truck/TruckMaker/Two_TRack_Model ==
  Mesurement : Inport
  Inputs : Inport  Port=2
  ACC_X : TruckMaker4SL/Read CM Dict  Commented=on  xname=Sensor.Inertial.Vhcl.VchBdy.Acc_B.x  xsync=off  xstime=Continuous
      settings: SourceProductName=TruckMaker4SL
  ACC_Y : TruckMaker4SL/Read CM Dict  Commented=on  xname=Sensor.Inertial.Vhcl.VchBdy.Acc_B.y  xsync=off  xstime=Continuous
      settings: SourceProductName=TruckMaker4SL
  Alpha : Scope  NumInputPorts=2
      settings: ActiveDisplayYMinimum=-0.063500444111812465  ActiveDisplayYMaximum=0.098419855798011671  DataLoggingVariableName=ScopeData5
  CP_vyFL : Scope  NumInputPorts=2
      settings: ActiveDisplayYMinimum=-0.85924840843530359  ActiveDisplayYMaximum=0.12983944400495923
  Constant1 : Constant  Commented=on  Value=0.01
  Demux : Demux  Outputs=7
  Demux1 : Demux  Commented=on  Outputs=2
  Demux2 : Demux  Outputs=2
  Demux3 : Demux  Outputs=2
  EKF_ONE_TRACK : MATLAB Function  Commented=on  TreatAsAtomicUnit=on
  Gain : Gain  Commented=on  Gain=0.5
  MATLAB Function : MATLAB Function  Commented=on  TreatAsAtomicUnit=on
  MATLAB Function1 : MATLAB Function  Commented=on  TreatAsAtomicUnit=on
  MATLAB Function2 : MATLAB Function  Commented=on  TreatAsAtomicUnit=on
  MATLAB Function3 : MATLAB Function  Commented=on  TreatAsAtomicUnit=on
  Mux : Mux  Commented=on  Inputs=5
  Mux1 : Mux  Commented=on  Inputs=2
  OMEGA_Z : TruckMaker4SL/Read CM Dict  Commented=on  xname=Car.YawRate  xsync=off  xstime=Continuous
      settings: SourceProductName=TruckMaker4SL
  Q : Constant  Value=diag([10 10 10 1e6 1e6])
  Q1 : Constant  Commented=on  Value=diag([1 1 1 1e5 1e5])
  Q2 : Constant  Value=diag([2 2 2 0 0 0 0 ]);
  Q_ : Constant  Commented=on  Value=diag([0.1, 0.1, 0.01])
  R : Constant  Value="diag([0.001 0.001  0.11 0.11  0.001   ]);"
  R1 : Constant  Commented=on  Value=diag([1 1 0.1 0.1 0.1 0.1 0.1]);
  R2 : Constant  Value=diag([0.2 0.2 0.1 0.1 0.001 3e-4 3e-3 3e-4 3e-4]);
  R_ : Constant  Commented=on  Value=diag([0.5 0.5 0.5 0.5 0.01 ])
  Read CM Dict : TruckMaker4SL/Read CM Dict  xname=Vhcl.FL.SideSlip  xsync=off  xstime=Continuous
      settings: SourceProductName=TruckMaker4SL
  Read CM Dict1 : TruckMaker4SL/Read CM Dict  xname=Car.vyFL  xsync=off  xstime=Continuous
      settings: SourceProductName=TruckMaker4SL
  Read CM Dict11 : TruckMaker4SL/Read CM Dict  Commented=on  xname=Car.SteerAngleFR  xsync=off  xstime=Continuous
      settings: SourceProductName=TruckMaker4SL
  Read CM Dict3 : TruckMaker4SL/Read CM Dict  Commented=on  xname=Vhcl.RL.Trq_Drive  xsync=off  xstime=Continuous
      settings: SourceProductName=TruckMaker4SL
  Read CM Dict6 : TruckMaker4SL/Read CM Dict  Commented=on  xname=Car.SteerAngleFL  xsync=off  xstime=Continuous
      settings: SourceProductName=TruckMaker4SL
  Read CM Dict8 : TruckMaker4SL/Read CM Dict  Commented=on  xname=Vhcl.RR.Trq_Drive  xsync=off  xstime=Continuous
      settings: SourceProductName=TruckMaker4SL
  ST : Constant  Value=0.01
  Scope : Scope  Commented=on
      settings: ActiveDisplayYMinimum=-478936.06463610154  ActiveDisplayYMaximum=-463543.54710663384  DataLoggingVariableName=ScopeData28
  Scope{1,4..7} (5 alike) : Scope
      Scope1 settings: ActiveDisplayYMinimum=0.29399310213887048  ActiveDisplayYMaximum=0.32573554644954378  DataLoggingVariableName=ScopeData7
      Scope4 settings: ActiveDisplayYMinimum=4.3726192136365007  ActiveDisplayYMaximum=40.865319844733996  DataLoggingVariableName=ScopeData38
      Scope5 settings: ActiveDisplayYMinimum=-1  ActiveDisplayYMaximum=1  DataLoggingVariableName=ScopeData39
      Scope6 settings: ActiveDisplayYMinimum=-1  ActiveDisplayYMaximum=1  DataLoggingVariableName=ScopeData42
      Scope7 settings: ActiveDisplayYMinimum=-1  ActiveDisplayYMaximum=1  DataLoggingVariableName=ScopeData43
  Scope2 : Scope  Commented=on
      settings: ActiveDisplayYMinimum=-1  ActiveDisplayYMaximum=1  DataLoggingVariableName=ScopeData8
  Scope3 : Scope  Commented=on
      settings: ActiveDisplayYMinimum=-339854.99447017239  ActiveDisplayYMaximum=-324915.14615423739  DataLoggingVariableName=ScopeData29
  Sensor_Vx : TruckMaker4SL/Read CM Dict  Commented=on  xname=Sensor.Inertial.Vhcl.VchBdy.Vel_B.x  xsync=off  xstime=Continuous
      settings: SourceProductName=TruckMaker4SL
  Sensor_Vy : TruckMaker4SL/Read CM Dict  Commented=on  xname=Sensor.Inertial.Vhcl.VchBdy.Vel_B.y  xsync=off  xstime=Continuous
      settings: SourceProductName=TruckMaker4SL
  Sum : Sum  Commented=on  Inputs=|++
  Terminator : Terminator  Commented=on
  Terminator1 : Terminator
  To Workspace : ToWorkspace  VariableName=xhat_two  SaveFormat=Timeseries  SampleTime=-1
  To Workspace1 : ToWorkspace  VariableName=Phat_two  SaveFormat=Timeseries  SampleTime=-1
  Ts : Constant  Commented=on  Value=0.01
  Two Track Model : MATLAB Function  TreatAsAtomicUnit=on  SystemSampleTime=0.01
  Two Track Model1 : MATLAB Function  Commented=on  TreatAsAtomicUnit=on
  UKF_ONE_TRACK : MATLAB Function  Commented=on  TreatAsAtomicUnit=on
  samplings time : Constant  Value=0.001
  vx : Outport
  vy : Outport  Port=2
  wz : Outport  Port=3
  CyFL : Outport  Port=4
  CyRL : Outport  Port=5
  CyRR : Outport  Port=6
  CyFR : Outport  Port=7
  wires:
  R/1 -> UKF_ONE_TRACK/2(u)
  Q/1 -> UKF_ONE_TRACK/3(Q)
  samplings time/1 -> UKF_ONE_TRACK/4(Ts)
  R1/1 -> EKF_ONE_TRACK/4(R)
  Q1/1 -> EKF_ONE_TRACK/3(Q)
  Constant1/1 -> EKF_ONE_TRACK/5(Ts)
  Demux3/1 -> Scope1/1
  Demux/3 -> wz/1
  Demux/2 -> vy/1
  Q_/1 -> ?
  R_/1 -> ?
  Ts/1 -> MATLAB Function2/3(Ts)
  Demux/4 -> Scope4/1, CyFL/1
  Demux/1 -> vx/1
  MATLAB Function2/6(Fyf) -> Scope2/1
  Two Track Model/2(P_out) -> To Workspace1/1, Terminator1/1
  MATLAB Function3/2(P) -> Terminator/1
  Mesurement/1 -> Two Track Model1/1(z), Two Track Model/1(z)
  Inputs/1 -> Two Track Model1/2(u), Two Track Model/2(u)
  Two Track Model/1(xhat) -> To Workspace/1, Demux/1  "State_estimates"
  ST/1 -> Two Track Model1/5(Ts), Two Track Model/5(Ts)
  R2/1 -> Two Track Model/4(R), Two Track Model1/4(R)
  Q2/1 -> Two Track Model1/3(Q), Two Track Model/3(Q)
  Two Track Model/3(Fy_mean) -> Demux3/1
  Two Track Model/4(alpha_mean) -> Demux2/1
  Demux2/1 -> Alpha/2
  Read CM Dict/1 -> Alpha/1
  Two Track Model/5(V_FL_whl) -> Demux1/1  "V_FL_WHL"
  Read CM Dict1/1 -> CP_vyFL/1
  Demux1/2 -> CP_vyFL/2
  Demux/5 -> Scope5/1, CyRL/1
  Sensor_Vx/1 -> Mux/3
  ACC_Y/1 -> Mux/2
  Sensor_Vy/1 -> Mux/4
  ACC_X/1 -> Mux/1
  OMEGA_Z/1 -> Mux/5  "omega_sensor"
  Mux/1 -> MATLAB Function2/1(z)
  Read CM Dict6/1 -> Sum/2
  Sum/1 -> Gain/1
  Read CM Dict11/1 -> Sum/1
  Read CM Dict3/1 -> Mux1/2
  Gain/1 -> Mux1/1
  Mux1/1 -> MATLAB Function2/2(u)
  MATLAB Function2/4(Cf_est) -> Scope/1
  MATLAB Function2/5(Cr_est) -> Scope3/1
  Demux/6 -> Scope6/1, CyRR/1
  Demux/7 -> Scope7/1, CyFR/1

== system generic_truck/TruckMaker/VehicleControl ==
  note: <Your model here>
  note: When implementing a vehicle control model,
      | be sure to add '-disablevehiclecontrol' to the command line arguments
      | in the CarMaker Model Configuration block.
      | Otherwise your model will possibly not see the original DrivMan signals
      | on its inputs, but those of a currently activated C-coded vehicle control model instead.
  Sync_In : Inport
  DrivMan.In : Inport  Port=2
  Bus Creator2 : BusCreator  Inputs=2
  CreateBus Vhcl.Misc : Subsystem
  CreateBus Vhcl.Wheel.In : Subsystem
  CreateBus VhclCtrl : Subsystem
  CreateBus VhclCtrl.PT : Subsystem
  CreateBus VhclCtrl.Steering : Subsystem
  Demux2 : Demux  Outputs=2
      settings: DisplayOption=none
  VehicleControl : S-Function  FunctionName=TM_Sfun  Parameters='VehicleControl'  SFunctionDeploymentMode=off  EnableBusSupport=off
  VehicleControlUpd : S-Function  FunctionName=TM_Sfun  Parameters='VehicleControlUpd'  SFunctionDeploymentMode=off  EnableBusSupport=off
  Sync_Out : Outport  VectorParamsAs1DForOutWhenUnconnected=off
  Vhcl.Model.Source : Outport  Port=2  VectorParamsAs1DForOutWhenUnconnected=off
  VhclCtrl.Steering : Outport  Port=3  VectorParamsAs1DForOutWhenUnconnected=off
  Vhcl.Wheel.In : Outport  Port=4  VectorParamsAs1DForOutWhenUnconnected=off
  Vhcl.Misc : Outport  Port=5  VectorParamsAs1DForOutWhenUnconnected=off
  VhclCtrl.Brake : Outport  Port=6  VectorParamsAs1DForOutWhenUnconnected=off
  VhclCtrl.PT : Outport  Port=7  VectorParamsAs1DForOutWhenUnconnected=off
  wires:
  VehicleControlUpd/2 -> Vhcl.Model.Source/1
  VehicleControlUpd/4 -> CreateBus Vhcl.Wheel.In/1(In1)
  VehicleControlUpd/5 -> CreateBus Vhcl.Misc/1(In1)
  VehicleControlUpd/6 -> Demux2/1
  VehicleControlUpd/7 -> CreateBus VhclCtrl.PT/1(In1)
  VehicleControlUpd/3 -> CreateBus VhclCtrl.Steering/1(In1)
  CreateBus Vhcl.Misc/1(Out1) -> Vhcl.Misc/1
  CreateBus Vhcl.Wheel.In/1(Out1) -> Vhcl.Wheel.In/1
  DrivMan.In/1 -> VehicleControl/2
  CreateBus VhclCtrl/1(Out) -> VehicleControlUpd/2
  VehicleControl/1 -> VehicleControlUpd/1
  VehicleControl/2 -> CreateBus VhclCtrl/1(In)
  Sync_In/1 -> VehicleControl/1
  CreateBus VhclCtrl.PT/1(Out1) -> VhclCtrl.PT/1
  Bus Creator2/1 -> VhclCtrl.Brake/1
  CreateBus VhclCtrl.Steering/1(Out1) -> VhclCtrl.Steering/1
  VehicleControlUpd/1 -> Sync_Out/1
  Demux2/2 -> Bus Creator2/2  "VhclCtrl BrakePark"
  Demux2/1 -> Bus Creator2/1  "VhclCtrl Brake"

== system generic_truck/TruckMaker/IPG Vehicle/Brake ==
  note: <Your model here>
  note: When replacing the entire braking system,
      | be sure to disable the IPG brake model by using the brake
      | model 'Model Manager off' in the vehicle GUI.
  Sync_In : Inport
  Brake.IF.In : Inport  Port=2
  VhclCtrl.Brake : Inport  Port=3
  Brake : S-Function  FunctionName=TM_Sfun  Parameters='Brake'  SFunctionDeploymentMode=off  EnableBusSupport=off
  BrakeUpd : S-Function  FunctionName=TM_Sfun  Parameters='BrakeUpd'  SFunctionDeploymentMode=off  EnableBusSupport=off
  BusCreator : BusCreator  Inputs=48
  CreateBus Vhcl.Wheel.PT : Subsystem
  Demux : Demux  Outputs=48
      settings: DisplayOption=none
  Sync_Out : Outport  VectorParamsAs1DForOutWhenUnconnected=off
  Vhcl.Wheel.PT : Outport  Port=2  VectorParamsAs1DForOutWhenUnconnected=off
  wires:
  Demux/1 -> BusCreator/1  "Brake IF Trq_WB FL"
  Demux/2 -> BusCreator/2  "Brake IF Trq_WB FR"
  Demux/3 -> BusCreator/3  "Brake IF Trq_WB RL"
  Demux/4 -> BusCreator/4  "Brake IF Trq_WB RR"
  Demux/5 -> BusCreator/5  "Brake IF Trq_WB RL2"
  Demux/6 -> BusCreator/6  "Brake IF Trq_WB RR2"
  Demux/7 -> BusCreator/7  "Brake IF Trq_WB FL2"
  Demux/8 -> BusCreator/8  "Brake IF Trq_WB FR2"
  Demux/9 -> BusCreator/9  "Brake IF Trq_WB RL3"
  Demux/10 -> BusCreator/10  "Brake IF Trq_WB RR3"
  Demux/11 -> BusCreator/11  "Brake IF Trq_WB RL4"
  Demux/12 -> BusCreator/12  "Brake IF Trq_WB RR4"
  Demux/13 -> BusCreator/13  "Brake IF Trq_PB FL"
  Demux/14 -> BusCreator/14  "Brake IF Trq_PB FR"
  Demux/15 -> BusCreator/15  "Brake IF Trq_PB RL"
  Demux/16 -> BusCreator/16  "Brake IF Trq_PB RR"
  Demux/17 -> BusCreator/17  "Brake IF Trq_PB RL2"
  Demux/18 -> BusCreator/18  "Brake IF Trq_PB RR2"
  Demux/19 -> BusCreator/19  "Brake IF Trq_PB FL2"
  Demux/20 -> BusCreator/20  "Brake IF Trq_PB FR2"
  Demux/21 -> BusCreator/21  "Brake IF Trq_PB RL3"
  Demux/22 -> BusCreator/22  "Brake IF Trq_PB RR3"
  Demux/23 -> BusCreator/23  "Brake IF Trq_PB RL4"
  Demux/24 -> BusCreator/24  "Brake IF Trq_PB RR4"
  Demux/25 -> BusCreator/25  "Brake IF Trq_Reg_trg FL"
  Demux/26 -> BusCreator/26  "Brake IF Trq_Reg_trg FR"
  Demux/27 -> BusCreator/27  "Brake IF Trq_Reg_trg RL"
  Demux/28 -> BusCreator/28  "Brake IF Trq_Reg_trg RR"
  Demux/29 -> BusCreator/29  "Brake IF Trq_Reg_trg RL2"
  Demux/30 -> BusCreator/30  "Brake IF Trq_Reg_trg RR2"
  Demux/31 -> BusCreator/31  "Brake IF Trq_Reg_trg FL2"
  Demux/32 -> BusCreator/32  "Brake IF Trq_Reg_trg FR2"
  Demux/33 -> BusCreator/33  "Brake IF Trq_Reg_trg RL3"
  Demux/34 -> BusCreator/34  "Brake IF Trq_Reg_trg RR3"
  Demux/35 -> BusCreator/35  "Brake IF Trq_Reg_trg RL4"
  Demux/36 -> BusCreator/36  "Brake IF Trq_Reg_trg RR4"
  Demux/37 -> BusCreator/37  "Brake IF Trq_DriveSrc_trg d0"
  Demux/38 -> BusCreator/38  "Brake IF Trq_DriveSrc_trg d1"
  Demux/39 -> BusCreator/39  "Brake IF Trq_DriveSrc_trg d2"
  Demux/40 -> BusCreator/40  "Brake IF Trq_DriveSrc_trg d3"
  Demux/41 -> BusCreator/41  "Brake IF Trq_DriveSrc_trg d4"
  Demux/42 -> BusCreator/42  "Brake IF Trq_DriveSrc_trg d5"
  Demux/43 -> BusCreator/43  "Brake IF Trq_DriveSrc_trg d6"
  Demux/44 -> BusCreator/44  "Brake IF Trq_DriveSrc_trg d7"
  Demux/45 -> BusCreator/45  "Brake IF Trq_DriveSrc_trg d8"
  Demux/46 -> BusCreator/46  "Brake IF Trq_DriveSrc_trg d9"
  Demux/47 -> BusCreator/47  "Brake IF Trq_DriveSrc_trg d10"
  Demux/48 -> BusCreator/48  "Brake IF Trq_DriveSrc_trg d11"
  BusCreator/1 -> BrakeUpd/2
  Brake/2 -> Demux/1
  BrakeUpd/1 -> Sync_Out/1
  Brake/1 -> BrakeUpd/1  "Sync"
  Brake.IF.In/1 -> Brake/2
  VhclCtrl.Brake/1 -> Brake/3
  Sync_In/1 -> Brake/1
  BrakeUpd/2 -> CreateBus Vhcl.Wheel.PT/1(In)
  CreateBus Vhcl.Wheel.PT/1(Out) -> Vhcl.Wheel.PT/1

== system generic_truck/TruckMaker/IPG Vehicle/CarAndTrailer ==
  Sync_In : Inport
  VhclCtrl.Steering : Inport  Port=2
  Vhcl.Wheel.In : Inport  Port=3
  Vhcl.Misc : Inport  Port=4
  CarAndTrailerUpd : Subsystem
  Forces : Subsystem
  Ground : Ground
  Kinematics : Subsystem
  Kinetics : Subsystem
  Steering : Subsystem
  Terminator : Terminator
  Terminator1 : Terminator
  Trailer : Subsystem
  Sync_Out : Outport  VectorParamsAs1DForOutWhenUnconnected=off
  Brake.IF.In : Outport  Port=2  VectorParamsAs1DForOutWhenUnconnected=off
  wires:
  Trailer/16(Vhcl.Wheel.RR4) -> CarAndTrailerUpd/16(Vhcl.Wheel.RR4)
  Trailer/15(Vhcl.Wheel.RL4) -> CarAndTrailerUpd/15(Vhcl.Wheel.RL4)
  Trailer/14(Vhcl.Wheel.RR3) -> CarAndTrailerUpd/14(Vhcl.Wheel.RR3)
  Trailer/13(Vhcl.Wheel.RL3) -> CarAndTrailerUpd/13(Vhcl.Wheel.RL3)
  Ground/1 -> CarAndTrailerUpd/18(Vhcl.Fr1A)
  Trailer/17(Car.Hitch.FrcTrq) -> CarAndTrailerUpd/17(Car.Hitch.FrcTrq)
  Trailer/12(Vhcl.Wheel.FR2) -> CarAndTrailerUpd/12(Vhcl.Wheel.FR2)
  Trailer/11(Vhcl.Wheel.FL2) -> CarAndTrailerUpd/11(Vhcl.Wheel.FL2)
  Trailer/10(Vhcl.Wheel.RR2) -> CarAndTrailerUpd/10(Vhcl.Wheel.RR2)
  Trailer/9(Vhcl.Wheel.RL2) -> CarAndTrailerUpd/9(Vhcl.Wheel.RL2)
  Trailer/8(Vhcl.Wheel.RR) -> CarAndTrailerUpd/8(Vhcl.Wheel.RR)
  Trailer/7(Vhcl.Wheel.RL) -> CarAndTrailerUpd/7(Vhcl.Wheel.RL)
  Trailer/6(Vhcl.Wheel.FR) -> CarAndTrailerUpd/6(Vhcl.Wheel.FR)
  Trailer/5(Vhcl.Wheel.FL) -> CarAndTrailerUpd/5(Vhcl.Wheel.FL)
  Trailer/4(Vhcl.PoI) -> CarAndTrailerUpd/4(Vhcl.PoI)
  Trailer/3(Vhcl.Motion) -> CarAndTrailerUpd/3(Vhcl.Motion)
  Trailer/2(Vhcl.Steering) -> CarAndTrailerUpd/2(Vhcl.Steering)
  Trailer/1(Sync_Out) -> CarAndTrailerUpd/1(Sync_In)
  CarAndTrailerUpd/2(Brake.IF.In) -> Brake.IF.In/1
  CarAndTrailerUpd/1(Sync_Out) -> Sync_Out/1
  Vhcl.Misc/1 -> Terminator1/1
  Vhcl.Wheel.In/1 -> Terminator/1
  Kinetics/6(WheelCarrier.Misc) -> Trailer/6(WheelCarrier.Misc)
  Kinetics/5(Car.Trq_T2W) -> Trailer/5(Car.Trq_T2W)
  Steering/2(Steer.IF) -> Kinematics/2(Steer.IF)
  Kinetics/4(Car.Fr1) -> Trailer/4(Car.Fr1)
  Kinetics/3(Car.Hitch) -> Trailer/3(Car.Hitch)
  Kinetics/2(Trailer.Load) -> Trailer/2(Trailer.Load)
  VhclCtrl.Steering/1 -> Steering/2(VhclCtrl.Steering)
  Sync_In/1 -> Steering/1(Sync_In)
  Steering/1(Sync_Out) -> Kinematics/1(Sync_In)
  Kinetics/1(Sync_Out) -> Trailer/1(Sync_In)
  Kinematics/5(lBuf) -> Forces/5(lBuf)
  Forces/4(Car.Load) -> Kinetics/4(Car.Load)
  Forces/2(Car.Virtual) -> Kinetics/2(Car.Virtual)
  Kinematics/2(lSpring) -> Forces/2(lSpring)
  Kinematics/3(vDamp) -> Forces/3(vDamp)
  Forces/3(Car.Aero) -> Kinetics/3(Car.Aero)
  Forces/1(Sync_Out) -> Kinetics/1(Sync_In)
  Kinematics/1(Sync_Out) -> Forces/1(Sync_In)
  Kinematics/4(lStabi) -> Forces/4(lStabi)
  Kinematics/6(tWheelCarrier_z) -> Forces/6(tWheelCarrier_z)
